simulink model "poprawiony_model_all_X2014_2n"  (R2014a)
settings: Solver=ode4  StartTime=0.0  StopTime=20  FixedStep=0.001  RelTol=1e-3
values from neighbouring files (symbols this model uses):
  A = [0 1 ... (first row only)    [cel.m]    (also in celPID.m; min_PID.m; pod_discPID.m; por_model_obiekt_osX.m)
  B = [0; k/omega0^2]    [cel.m]    (also in celPID.m; min_PID.m; pod_discPID.m; por_model_obiekt_osX.m)
  C = [1 0]    [cel.m]    (also in celPID.m; min_PID.m; pod_discPID.m; por_model_obiekt_osX.m)
  D = 0    [cel.m]    (also in celPID.m; min_PID.m; pod_discPID.m; por_model_obiekt_osX.m)
  Dr = X(5)    [celPID.m]    (also in min_PID.m = 2; pod_discPID.m = 2)
  Dx = X(2)    [celPID.m]    (also in dane.m = 0.01; min_PID.m = 0.01; pod_discPID.m = 0.01)
  Ir = X(4)    [celPID.m]    (also in min_PID.m = 0.005; pod_discPID.m = 0.005)
  KT = -1/32    (= -0.03125)    [celPID.m]    (also in min_PID.m; pod_discPID.m; por_model_obiekt_osX.m; por_model_obiekt_osY.m)
  limitT = 0.05    [cel.m]    (also in celPID.m; dane.m; pod_discPID.m)
  omega = 4.37    [cel.m]    (also in celPID.m = 0.228832951945; dane.m = 0.222816399287; min_PID.m = 0.231; pod_discPID.m = 0.228832951945)
  Pdx = X(1)    [celPID.m]    (also in dane.m = 10; min_PID.m = 10; pod_discPID.m = 10)
  Pr = X(3)    [celPID.m]    (also in min_PID.m = 10; pod_discPID.m = 10)
  reg_PD = -1    [celPID.m]    (also in dane.m; min_PID.m; pod_discPID.m)
  X0 = [0 0 0 0]    [cel.m]    (also in celPID.m = [0 0]; min_PID.m = [0 0]; pod_discPID.m = [0 0]; por_model_obiekt_osX.m = [0 0])
  x0 = [0   0   0    0   0   0    0   0   0.50   0]'    [dane.m]
libraries: simulink x4
settings Model: CovModelRefEnable=off  CovSFcnEnable=on  Creator=Maciek  LastModifiedBy=Maciek
settings DataIOCC: LimitDataPoints=off  SaveFormat=StructureWithTime
settings DebuggingCC: MergeDetectMultiDrivingBlocksExec=error  SolverPrmCheckMsg=none  FrameProcessingCompatibilityMsg=error
settings HardwareCC: ProdBitPerPointer=64  ProdLargestAtomicFloat=Float  ProdIntDivRoundTo=Zero  ProdEndianess=LittleEndian  ProdHWDeviceType=Specified
settings ModelReferenceCC: PropagateSignalLabelsOutOfModel=on

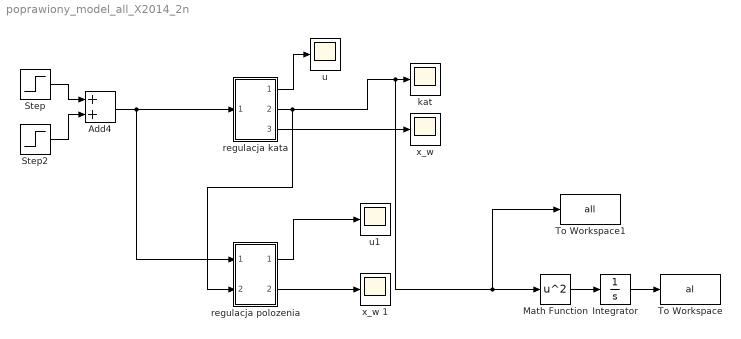
== system poprawiony_model_all_X2014_2n ==
  Add4 : Sum
  Integrator : Integrator
  Math Function : Math  Operator=square  SaturateOnIntegerOverflow=on
  Step : Step  After=0.2  SampleTime=0
  Step2 : Step  Time=40  After=-0.7  SampleTime=0
  To Workspace : ToWorkspace  VariableName=al  SaveFormat=Timeseries  SampleTime=-1
      settings: MaxDataPoints=1
  To Workspace1 : ToWorkspace  VariableName=all  SaveFormat=Timeseries  SampleTime=-1
  kat : Scope
      settings: TimeRange=auto  MaxDataPoints=5000  SaveName=kat  YMin=-0.08187  YMax=0.08063  SampleTime=-1
  regulacja kata : Subsystem
  regulacja polozenia : Subsystem
  u : Scope
      settings: TimeRange=auto  MaxDataPoints=5000  SaveName=ScopeData4  YMin=-1.25  YMax=1.25  SampleTime=-1
  u1 : Scope
      settings: TimeRange=auto  MaxDataPoints=5000  SaveName=ScopeData5  YMin=-0.125  YMax=1.125  SampleTime=-1
  "x_w " : Scope
      settings: TimeRange=auto  MaxDataPoints=5000  SaveName=ScopeData6  YMin=-0.02566  YMax=0.23098  SampleTime=-1
  x_w 1 : Scope
      settings: TimeRange=auto  MaxDataPoints=5000  SaveName=x  YMin=-0.02653  YMax=0.23778  SampleTime=-1
  wires:
  Step/1 -> Add4/1
  Step2/1 -> Add4/2
  regulacja kata/1(Out1) -> u/1
  regulacja kata/2(Out2) -> regulacja polozenia/2(kat), To Workspace1/1, Math Function/1, kat/1
  regulacja kata/3(Out3) -> "x_w "/1
  Add4/1 -> regulacja polozenia/1(In1), regulacja kata/1(In1)
  regulacja polozenia/1(Out1) -> u1/1
  Math Function/1 -> Integrator/1
  Integrator/1 -> To Workspace/1
  regulacja polozenia/2(Out3) -> x_w 1/1

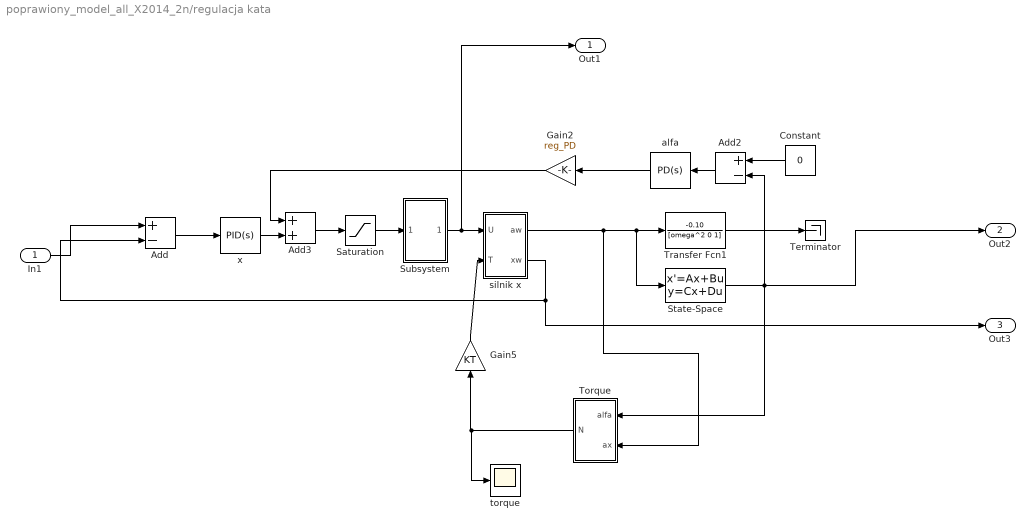
== system poprawiony_model_all_X2014_2n/regulacja kata ==
  In1 : Inport
  Add : Sum  Inputs=+-
  Add2 : Sum  Inputs=+-
  Add3 : Sum
  Constant : Constant  Value=0
  Gain2 : Gain  Gain=reg_PD
  Gain5 : Gain  Gain=KT
  Saturation : Saturate  UpperLimit=1  LowerLimit=-1
  State-Space : StateSpace  A=A  B=B  C=C  D=D  X0=X0
  Subsystem : Subsystem
  Terminator : Terminator
  "Torque " : Subsystem
  Transfer Fcn1 : TransferFcn  Numerator=-0.10  Denominator=[omega^2 0 1]
  alfa : simulink/Continuous/PID Controller  Controller=PD  TimeDomain=Continuous-time  SampleTime=-1  IntegratorMethod=Forward Euler  FilterMethod=Forward Euler  Form=Parallel  UseFilter=on  ControllerParametersSource=internal  P=Pdx  I=0.015  D=Dx  N=100  InitialConditionSource=internal  InitialConditionForIntegrator=0  InitialConditionForFilter=0  ExternalReset=none  LimitOutput=on  UpperSaturationLimit=1  LowerSaturationLimit=-1  LinearizeAsGain=on  AntiWindupMode=none  Kb=1  TrackingMode=off  Kt=1  PParamMin=[]  PParamMax=[]  IParamMin=[]  IParamMax=[]  DParamMin=[]  DParamMax=[]  NParamMin=[]  NParamMax=[]  KbParamMin=[]  KbParamMax=[]  KtParamMin=[]  KtParamMax=[]  POutMin=[]  POutMax=[]  IOutMin=[]  IOutMax=[]  DOutMin=[]  DOutMax=[]  NOutMin=[]  NOutMax=[]  KbOutMin=[]  KbOutMax=[]  KtOutMin=[]  KtOutMax=[]  IntegratorOutMin=[]  IntegratorOutMax=[]  FilterOutMin=[]  FilterOutMax=[]  SumOutMin=[]  SumOutMax=[]  SumI1OutMin=[]  SumI1OutMax=[]  SumI2OutMin=[]  SumI2OutMax=[]  SumI3OutMin=[]  SumI3OutMax=[]  SumDOutMin=[]  SumDOutMax=[]  SaturationOutMin=[]  SaturationOutMax=[]  IntegratorContinuousStateAttributes=''  IntegratorStateMustResolveToSignalObject=off  IntegratorRTWStateStorageClass=Auto  FilterContinuousStateAttributes=''  FilterStateMustResolveToSignalObject=off  FilterRTWStateStorageClass=Auto  DifferentiatorICPrevScaledInput=0  DifferentiatorOutMin=[]  DifferentiatorOutMax=[]
  silnik x : Subsystem
  torque : Scope
      settings: TimeRange=auto  LimitDataPoints=on  MaxDataPoints=5000  SaveToWorkspace=off  SaveName=ScopeData3  YMin=-10  YMax=10  SampleTime=-1  DataFormat=Array
  x : simulink/Continuous/PID Controller  Controller=PID  TimeDomain=Continuous-time  SampleTime=-1  IntegratorMethod=Forward Euler  FilterMethod=Forward Euler  Form=Parallel  UseFilter=on  ControllerParametersSource=internal  P=Pr  I=Ir  D=Dr  N=100  InitialConditionSource=internal  InitialConditionForIntegrator=0  InitialConditionForFilter=0  ExternalReset=none  LimitOutput=on  UpperSaturationLimit=1  LowerSaturationLimit=-1  LinearizeAsGain=on  AntiWindupMode=none  Kb=1  TrackingMode=off  Kt=1  PParamMin=[]  PParamMax=[]  IParamMin=[]  IParamMax=[]  DParamMin=[]  DParamMax=[]  NParamMin=[]  NParamMax=[]  KbParamMin=[]  KbParamMax=[]  KtParamMin=[]  KtParamMax=[]  POutMin=[]  POutMax=[]  IOutMin=[]  IOutMax=[]  DOutMin=[]  DOutMax=[]  NOutMin=[]  NOutMax=[]  KbOutMin=[]  KbOutMax=[]  KtOutMin=[]  KtOutMax=[]  IntegratorOutMin=[]  IntegratorOutMax=[]  FilterOutMin=[]  FilterOutMax=[]  SumOutMin=[]  SumOutMax=[]  SumI1OutMin=[]  SumI1OutMax=[]  SumI2OutMin=[]  SumI2OutMax=[]  SumI3OutMin=[]  SumI3OutMax=[]  SumDOutMin=[]  SumDOutMax=[]  SaturationOutMin=[]  SaturationOutMax=[]  IntegratorContinuousStateAttributes=''  IntegratorStateMustResolveToSignalObject=off  IntegratorRTWStateStorageClass=Auto  FilterContinuousStateAttributes=''  FilterStateMustResolveToSignalObject=off  FilterRTWStateStorageClass=Auto  DifferentiatorICPrevScaledInput=0  DifferentiatorOutMin=[]  DifferentiatorOutMax=[]
  Out1 : Outport
  Out2 : Outport  Port=2
  Out3 : Outport  Port=3
  wires:
  Add/1 -> x/1
  Add2/1 -> alfa/1
  Constant/1 -> Add2/1
  alfa/1 -> Gain2/1
  x/1 -> Add3/2
  Gain2/1 -> Add3/1
  silnik x/1(aw) -> "Torque "/2(ax), State-Space/1, Transfer Fcn1/1
  In1/1 -> Add/1
  Add3/1 -> Saturation/1
  Gain5/1 -> silnik x/2(T)
  "Torque "/1(N) -> Gain5/1, torque/1
  State-Space/1 -> "Torque "/1(alfa), Add2/2, Out2/1
  Transfer Fcn1/1 -> Terminator/1
  silnik x/2(xw) -> Out3/1, Add/2
  Subsystem/1(Out1) -> Out1/1, silnik x/1(U)
  Saturation/1 -> Subsystem/1(In1)

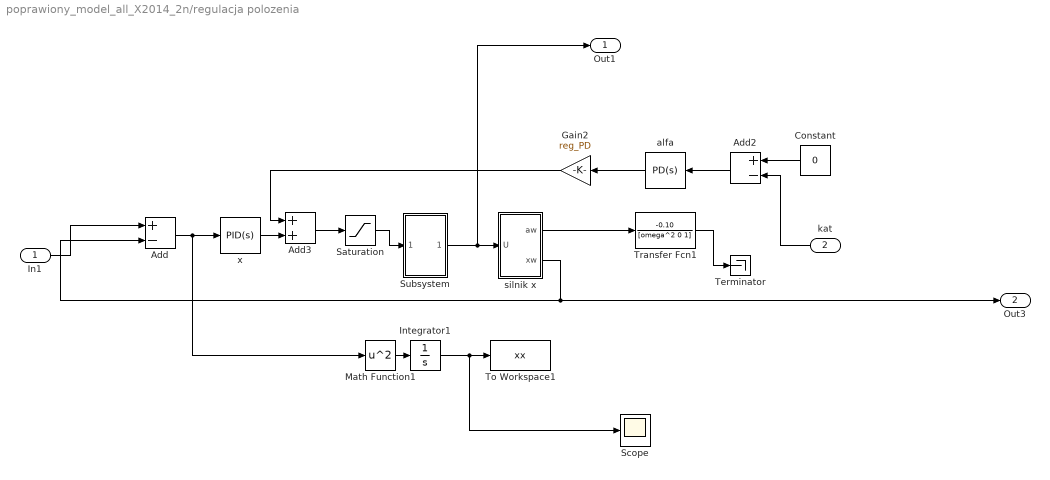
== system poprawiony_model_all_X2014_2n/regulacja polozenia ==
  In1 : Inport
  kat : Inport  Port=2
  Add : Sum  Inputs=+-
  Add2 : Sum  Inputs=+-
  Add3 : Sum
  Constant : Constant  Value=0
  Gain2 : Gain  Gain=reg_PD
  Integrator1 : Integrator
  Math Function1 : Math  Operator=square  SaturateOnIntegerOverflow=on
  Saturation : Saturate  UpperLimit=1  LowerLimit=-1
  Scope : Scope
      settings: TimeRange=auto  MaxDataPoints=5000  SaveToWorkspace=off  SaveName=ScopeData  YMin=-0.00467  YMax=0.04201  SampleTime=-1
  Subsystem : Subsystem
  Terminator : Terminator
  To Workspace1 : ToWorkspace  VariableName=xx  SaveFormat=Timeseries  SampleTime=-1
      settings: MaxDataPoints=1
  Transfer Fcn1 : TransferFcn  Numerator=-0.10  Denominator=[omega^2 0 1]
  alfa : simulink/Continuous/PID Controller  Controller=PD  TimeDomain=Continuous-time  SampleTime=-1  IntegratorMethod=Forward Euler  FilterMethod=Forward Euler  Form=Parallel  UseFilter=on  ControllerParametersSource=internal  P=Pdx  I=0.015  D=Dx  N=100  InitialConditionSource=internal  InitialConditionForIntegrator=0  InitialConditionForFilter=0  ExternalReset=none  LimitOutput=on  UpperSaturationLimit=1  LowerSaturationLimit=-1  LinearizeAsGain=on  AntiWindupMode=none  Kb=1  TrackingMode=off  Kt=1  PParamMin=[]  PParamMax=[]  IParamMin=[]  IParamMax=[]  DParamMin=[]  DParamMax=[]  NParamMin=[]  NParamMax=[]  KbParamMin=[]  KbParamMax=[]  KtParamMin=[]  KtParamMax=[]  POutMin=[]  POutMax=[]  IOutMin=[]  IOutMax=[]  DOutMin=[]  DOutMax=[]  NOutMin=[]  NOutMax=[]  KbOutMin=[]  KbOutMax=[]  KtOutMin=[]  KtOutMax=[]  IntegratorOutMin=[]  IntegratorOutMax=[]  FilterOutMin=[]  FilterOutMax=[]  SumOutMin=[]  SumOutMax=[]  SumI1OutMin=[]  SumI1OutMax=[]  SumI2OutMin=[]  SumI2OutMax=[]  SumI3OutMin=[]  SumI3OutMax=[]  SumDOutMin=[]  SumDOutMax=[]  SaturationOutMin=[]  SaturationOutMax=[]  IntegratorContinuousStateAttributes=''  IntegratorStateMustResolveToSignalObject=off  IntegratorRTWStateStorageClass=Auto  FilterContinuousStateAttributes=''  FilterStateMustResolveToSignalObject=off  FilterRTWStateStorageClass=Auto  DifferentiatorICPrevScaledInput=0  DifferentiatorOutMin=[]  DifferentiatorOutMax=[]
  silnik x : Subsystem
  x : simulink/Continuous/PID Controller  Controller=PID  TimeDomain=Continuous-time  SampleTime=-1  IntegratorMethod=Forward Euler  FilterMethod=Forward Euler  Form=Parallel  UseFilter=on  ControllerParametersSource=internal  P=Pr  I=Ir  D=Dr  N=100  InitialConditionSource=internal  InitialConditionForIntegrator=0  InitialConditionForFilter=0  ExternalReset=none  LimitOutput=on  UpperSaturationLimit=1  LowerSaturationLimit=-1  LinearizeAsGain=on  AntiWindupMode=none  Kb=1  TrackingMode=off  Kt=1  PParamMin=[]  PParamMax=[]  IParamMin=[]  IParamMax=[]  DParamMin=[]  DParamMax=[]  NParamMin=[]  NParamMax=[]  KbParamMin=[]  KbParamMax=[]  KtParamMin=[]  KtParamMax=[]  POutMin=[]  POutMax=[]  IOutMin=[]  IOutMax=[]  DOutMin=[]  DOutMax=[]  NOutMin=[]  NOutMax=[]  KbOutMin=[]  KbOutMax=[]  KtOutMin=[]  KtOutMax=[]  IntegratorOutMin=[]  IntegratorOutMax=[]  FilterOutMin=[]  FilterOutMax=[]  SumOutMin=[]  SumOutMax=[]  SumI1OutMin=[]  SumI1OutMax=[]  SumI2OutMin=[]  SumI2OutMax=[]  SumI3OutMin=[]  SumI3OutMax=[]  SumDOutMin=[]  SumDOutMax=[]  SaturationOutMin=[]  SaturationOutMax=[]  IntegratorContinuousStateAttributes=''  IntegratorStateMustResolveToSignalObject=off  IntegratorRTWStateStorageClass=Auto  FilterContinuousStateAttributes=''  FilterStateMustResolveToSignalObject=off  FilterRTWStateStorageClass=Auto  DifferentiatorICPrevScaledInput=0  DifferentiatorOutMin=[]  DifferentiatorOutMax=[]
  Out1 : Outport
  Out3 : Outport  Port=2
  wires:
  Add/1 -> Math Function1/1, x/1
  Add2/1 -> alfa/1
  Constant/1 -> Add2/1
  alfa/1 -> Gain2/1
  x/1 -> Add3/2
  Gain2/1 -> Add3/1
  silnik x/1(aw) -> Transfer Fcn1/1
  silnik x/2(xw) -> Out3/1, Add/2
  In1/1 -> Add/1
  Add3/1 -> Saturation/1
  kat/1 -> Add2/2
  Transfer Fcn1/1 -> Terminator/1
  Integrator1/1 -> Scope/1, To Workspace1/1
  Math Function1/1 -> Integrator1/1
  Subsystem/1(Out1) -> Out1/1, silnik x/1(U)
  Saturation/1 -> Subsystem/1(In1)

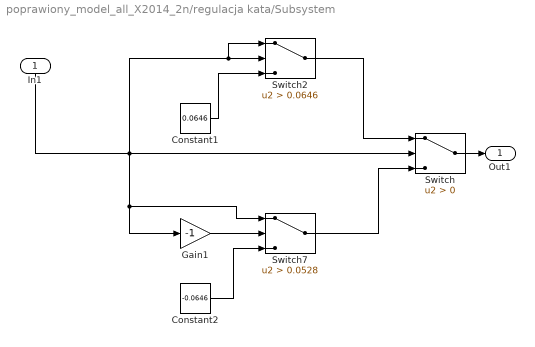
== system poprawiony_model_all_X2014_2n/regulacja kata/Subsystem ==
  In1 : Inport
  Constant1 : Constant  Value=0.0646
  Constant2 : Constant  Value=-0.0646
  Gain1 : Gain  Gain=-1
  Switch : Switch  Criteria=u2 > Threshold
  Switch2 : Switch  Criteria=u2 > Threshold  Threshold=0.0646
  Switch7 : Switch  Criteria=u2 > Threshold  Threshold=0.0528
  Out1 : Outport
  wires:
  In1/1 -> Switch7/1, Gain1/1, Switch2/1, Switch2/2, Switch/2
  Switch/1 -> Out1/1
  Constant1/1 -> Switch2/3
  Switch2/1 -> Switch/1
  Constant2/1 -> Switch7/3
  Gain1/1 -> Switch7/2
  Switch7/1 -> Switch/3

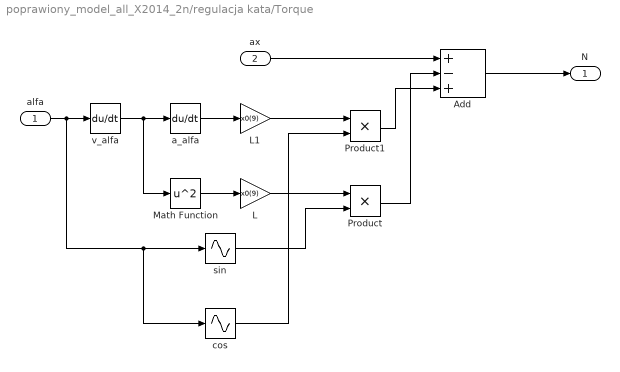
== system poprawiony_model_all_X2014_2n/regulacja kata/Torque  ==
  alfa : Inport
  ax : Inport  Port=2
  Add : Sum  Inputs=+-+
  L : Gain  Gain=x0(9)
  "L1 " : Gain  Gain=x0(9)
  Math Function : Math  Operator=square  SaturateOnIntegerOverflow=on
  Product : Product
  Product1 : Product
  a_alfa : Derivative
  cos : Sin  TimeSource=Use external signal  Phase=pi/2  SampleTime=0
  sin : Sin  TimeSource=Use external signal  SampleTime=0
  v_alfa : Derivative
  N : Outport
  wires:
  a_alfa/1 -> "L1 "/1
  v_alfa/1 -> Math Function/1, a_alfa/1
  Math Function/1 -> L/1
  L/1 -> Product/1
  Product/1 -> Add/2
  alfa/1 -> cos/1, sin/1, v_alfa/1
  "L1 "/1 -> Product1/1
  Product1/1 -> Add/3
  Add/1 -> N/1
  cos/1 -> Product1/2
  ax/1 -> Add/1
  sin/1 -> Product/2

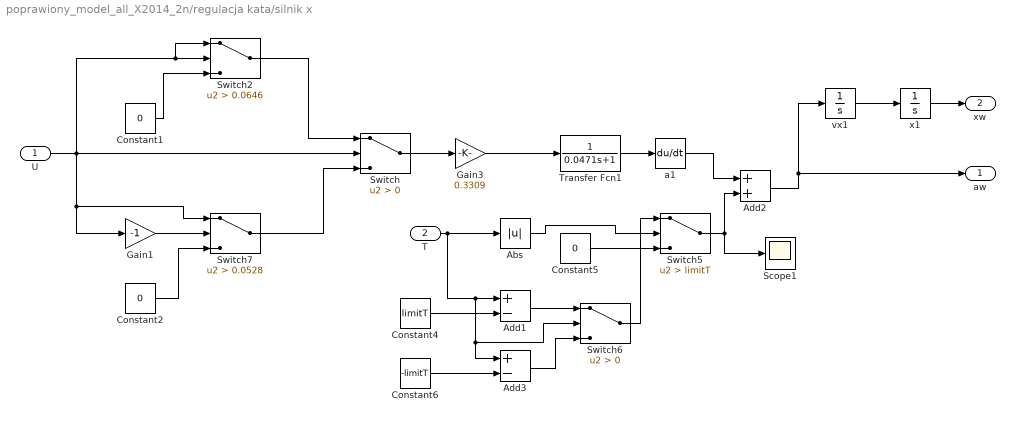
== system poprawiony_model_all_X2014_2n/regulacja kata/silnik x ==
  U : Inport
  T : Inport  Port=2
  Abs : Abs
  Add1 : Sum  Inputs=+-
  Add2 : Sum
  Add3 : Sum  Inputs=+-
  Constant1 : Constant  Value=0
  Constant2 : Constant  Value=0
  Constant4 : Constant  Value=limitT
  Constant5 : Constant  Value=0
  Constant6 : Constant  Value=-limitT
  Gain1 : Gain  Gain=-1
  Gain3 : Gain  Gain=0.3309
  Scope1 : Scope
      settings: TimeRange=auto  MaxDataPoints=5000  SaveToWorkspace=off  SaveName=ScopeData2  YMin=-0.45032  YMax=0.28533  SampleTime=-1
  Switch : Switch  Criteria=u2 > Threshold
  Switch2 : Switch  Criteria=u2 > Threshold  Threshold=0.0646
  Switch5 : Switch  Criteria=u2 > Threshold  Threshold=limitT
  Switch6 : Switch  Criteria=u2 > Threshold
  Switch7 : Switch  Criteria=u2 > Threshold  Threshold=0.0528
  Transfer Fcn1 : TransferFcn  Numerator=1  Denominator=[0.0471 1]
  a1 : Derivative
  vx1 : Integrator
  x1 : Integrator
  aw : Outport
  xw : Outport  Port=2
  wires:
  Constant1/1 -> Switch2/3
  Switch2/1 -> Switch/1
  Constant2/1 -> Switch7/3
  U/1 -> Switch7/1, Gain1/1, Switch2/1, Switch2/2, Switch/2
  Switch7/1 -> Switch/3
  Gain1/1 -> Switch7/2
  Transfer Fcn1/1 -> a1/1
  x1/1 -> xw/1
  vx1/1 -> x1/1
  Gain3/1 -> Transfer Fcn1/1
  Add2/1 -> aw/1, vx1/1
  a1/1 -> Add2/1
  Switch5/1 -> Scope1/1, Add2/2
  T/1 -> Add3/1, Switch6/2, Add1/1, Abs/1
  Abs/1 -> Switch5/2
  Constant4/1 -> Add1/2
  Constant5/1 -> Switch5/3
  Switch6/1 -> Switch5/1
  Add1/1 -> Switch6/1
  Constant6/1 -> Add3/2
  Add3/1 -> Switch6/3
  Switch/1 -> Gain3/1

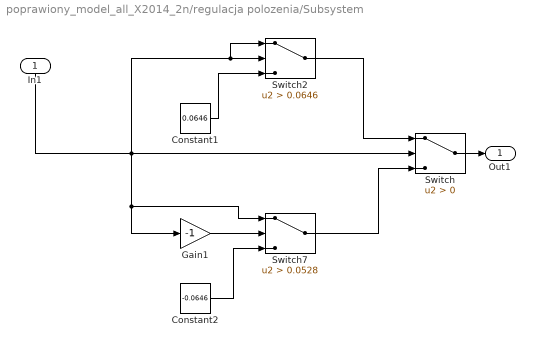
== system poprawiony_model_all_X2014_2n/regulacja polozenia/Subsystem ==
  In1 : Inport
  Constant1 : Constant  Value=0.0646
  Constant2 : Constant  Value=-0.0646
  Gain1 : Gain  Gain=-1
  Switch : Switch  Criteria=u2 > Threshold
  Switch2 : Switch  Criteria=u2 > Threshold  Threshold=0.0646
  Switch7 : Switch  Criteria=u2 > Threshold  Threshold=0.0528
  Out1 : Outport
  wires:
  In1/1 -> Switch7/1, Gain1/1, Switch2/1, Switch2/2, Switch/2
  Switch/1 -> Out1/1
  Constant1/1 -> Switch2/3
  Switch2/1 -> Switch/1
  Constant2/1 -> Switch7/3
  Gain1/1 -> Switch7/2
  Switch7/1 -> Switch/3

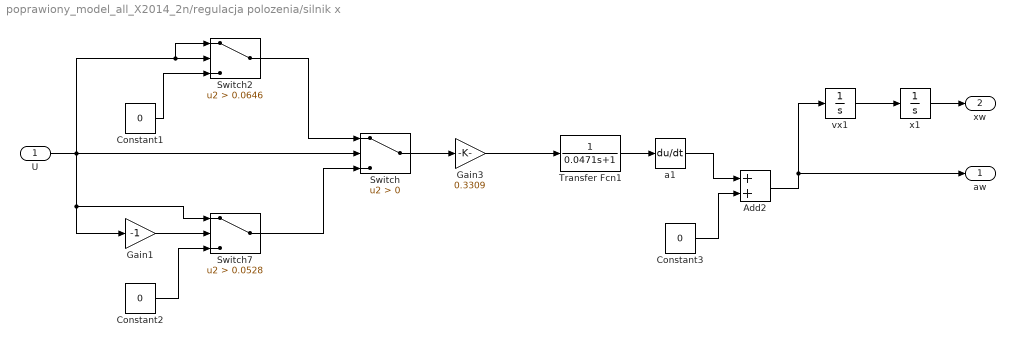
== system poprawiony_model_all_X2014_2n/regulacja polozenia/silnik x ==
  U : Inport
  Add2 : Sum
  Constant1 : Constant  Value=0
  Constant2 : Constant  Value=0
  Constant3 : Constant  Value=0
  Gain1 : Gain  Gain=-1
  Gain3 : Gain  Gain=0.3309
  Switch : Switch  Criteria=u2 > Threshold
  Switch2 : Switch  Criteria=u2 > Threshold  Threshold=0.0646
  Switch7 : Switch  Criteria=u2 > Threshold  Threshold=0.0528
  Transfer Fcn1 : TransferFcn  Numerator=1  Denominator=[0.0471 1]
  a1 : Derivative
  vx1 : Integrator
  x1 : Integrator
  aw : Outport
  xw : Outport  Port=2
  wires:
  Constant1/1 -> Switch2/3
  Switch2/1 -> Switch/1
  Constant2/1 -> Switch7/3
  U/1 -> Switch7/1, Gain1/1, Switch2/1, Switch2/2, Switch/2
  Switch7/1 -> Switch/3
  Gain1/1 -> Switch7/2
  Transfer Fcn1/1 -> a1/1
  x1/1 -> xw/1
  vx1/1 -> x1/1
  Gain3/1 -> Transfer Fcn1/1
  Add2/1 -> aw/1, vx1/1
  a1/1 -> Add2/1
  Switch/1 -> Gain3/1
  Constant3/1 -> Add2/2
